simulink model "doubleIt"  (R2020b)
settings: Solver=VariableStepAuto  StartTime=0.0  StopTime=0.5  FixedStep=1e4  RelTol=1e-3
settings Model: Creator=Kasper Laustsen  LastModifiedBy=Kasper Laustsen
settings SFSimCC: SimCustomHeaderCode="#include \"doubleIt.h\""  SimUserSources=doubleIt.c

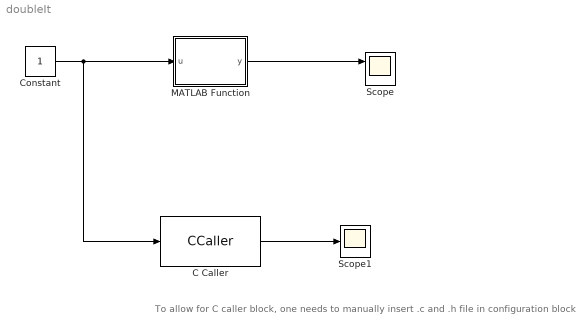
== system doubleIt ==
  note: To allow for C caller block, one needs to manually insert .c and .h file in configuration block
  C Caller : CCaller  FunctionName=doubleIt  PortSpecificationStruct="%)30     .    N ,   8    (     @         %    \"     (    !     0         %  0 \"0    $    _    07)G3F%M90  4&]R=$YA;64 4V-O<&4     26YD97@     5'EP90      4VEZ90      27-';&]B86P   X    P    !@    @    $          4    (     0    ,    !         !   P!O=70 #@   #     &    \"     0         !0    @    !     P    $         $  # &]U=  .    .     8    (    !          %    \"     $    &     0         0    !@   $]U='!U=   #@   #@    &    \"     8         !0    @    !     0    $         \"0    @               X    X    !@    @    $          4    (     0    8    !         !     &    9&]U8FQE   .    ,     8    (    !          %    \"     $    !     0         0  $ ,0    X    P    !@    @    ) @        4    (     0    $    !          (  0      #@   #     &    \"     0         !0    @    !     0    $         $  ! '4    .    ,     8    (    !          %    \"     $    !     0         0  $ =0    X    X    !@    @    $          4    (     0    4    !         !     %    26YP=70    .    .     8    (    !@         %    \"     $    !     0         )    \"               #@   #@    &    \"     0         !0    @    !    !@    $         $     8   !D;W5B;&4   X    P    !@    @    $          4    (     0    $    !         !   0 Q    #@   #     &    \"     D\"        !0    @    !     0    $          @ !"
  Constant : Constant
  MATLAB Function : MATLAB Function  TreatAsAtomicUnit=on
  Scope : Scope  NumInputPorts=2
  Scope1 : Scope
  wires:
  Constant/1 -> C Caller/1, MATLAB Function/1(u)
  MATLAB Function/1(y) -> Scope/1
  C Caller/1 -> Scope1/1

== matlab function doubleIt/MATLAB Function ==
  data: u input; y output
function y = callingDoubleIt(u)
% coder.updateBuildInfo('addSourceFiles','doubleIt.c');
% coder.cinclude('doubleIt.h');

y = 0.0;


y = coder.ceval('doubleIt',u);
